simulink model "run_bota_ethercat"  (R2021b)
settings: Solver=ode5  StartTime=0.0  StopTime=inf  FixedStep=0.001  RelTol=1e-3
settings Model: Creator=Martin Wermelinger  LastModifiedBy=Martin Wermelinger
settings CodeAppCC: MaxIdLength=95

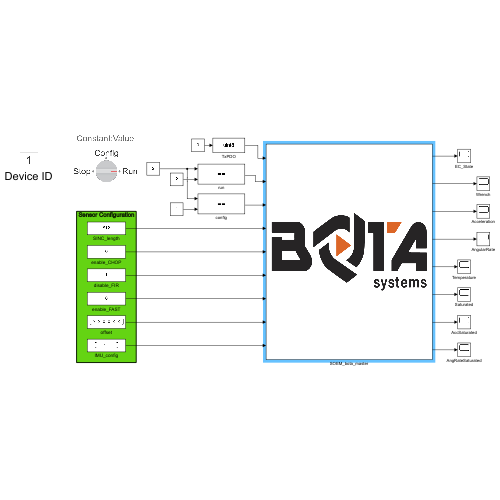
[thumbnail: Simulink's stored preview of the top-level diagram]
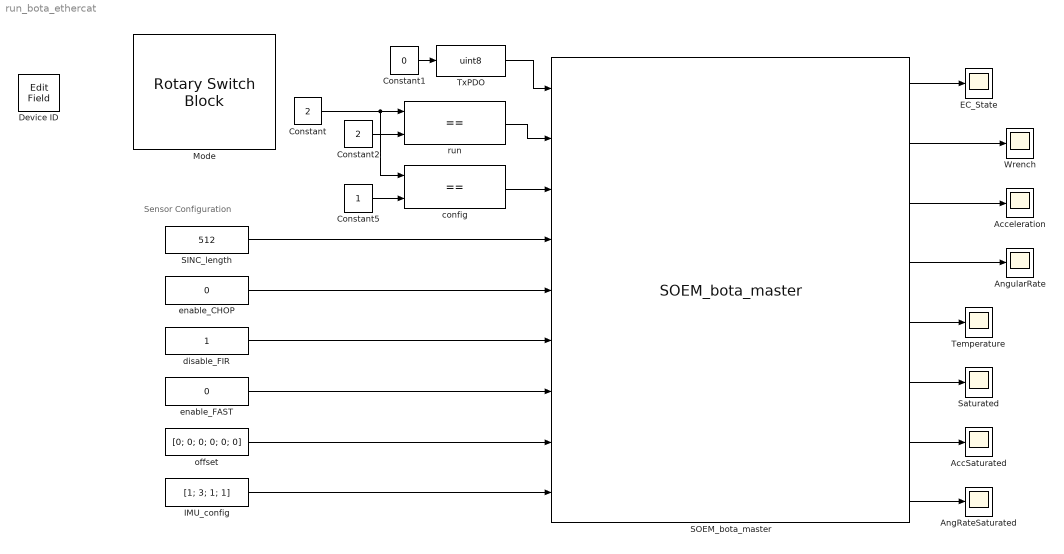
== system run_bota_ethercat ==
  note: Sensor Configuration
  AccSaturated : Scope
  Acceleration : Scope
  AngRateSaturated : Scope
  AngularRate : Scope
  Constant : Constant  Value=2  SampleTime=-1
  Constant1 : Constant  Value=0  SampleTime=0.001
  Constant2 : Constant  Value=2  SampleTime=-1
  Constant5 : Constant  SampleTime=-1
  Device ID : EditField  LabelPosition=Hide  ShowInitialText=on  Alignment=Center
  EC_State : Scope
  IMU_config : Constant  Value=[1; 3; 1; 1]  OutDataTypeStr=int8  SampleTime=-1
  Mode : RotarySwitchBlock
      settings: Values={{'Stop', 'Config', 'Run'}, [-1 1 2]}
  SINC_length : Constant  Value=512  OutDataTypeStr=uint16  SampleTime=-1
  SOEM_bota_master : S-Function  FunctionName=SOEM_bota_master  Parameters=1  SFunctionDeploymentMode=off  EnableBusSupport=off
      mask Display: image('$imagefile'); % Use "Edit Image" on toolstrip to change.
  Saturated : Scope
  Temperature : Scope
  TxPDO : DataTypeConversion  OutDataTypeStr=uint8
  Wrench : Scope
  config : RelationalOperator  Operator===  OutDataTypeStr=boolean  RndMeth=Simplest
  disable_FIR : Constant  OutDataTypeStr=uint8  SampleTime=-1
  enable_CHOP : Constant  Value=0  OutDataTypeStr=uint8  SampleTime=-1
  enable_FAST : Constant  Value=0  OutDataTypeStr=uint8  SampleTime=-1
  offset : Constant  Value=[0; 0; 0; 0; 0; 0]  OutDataTypeStr=single  SampleTime=-1
  run : RelationalOperator  Operator===  OutDataTypeStr=boolean  RndMeth=Simplest
  wires:
  IMU_config/1 -> SOEM_bota_master/9
  TxPDO/1 -> SOEM_bota_master/1
  SOEM_bota_master/1 -> EC_State/1
  offset/1 -> SOEM_bota_master/8
  Constant/1 -> config/1, run/1
  SOEM_bota_master/4 -> AngularRate/1
  SOEM_bota_master/8 -> AngRateSaturated/1
  SOEM_bota_master/7 -> AccSaturated/1
  SOEM_bota_master/6 -> Saturated/1
  SOEM_bota_master/5 -> Temperature/1
  Constant1/1 -> TxPDO/1
  SOEM_bota_master/3 -> Acceleration/1
  run/1 -> SOEM_bota_master/2
  Constant5/1 -> config/2
  disable_FIR/1 -> SOEM_bota_master/6
  enable_CHOP/1 -> SOEM_bota_master/5
  config/1 -> SOEM_bota_master/3
  SINC_length/1 -> SOEM_bota_master/4
  enable_FAST/1 -> SOEM_bota_master/7
  Constant2/1 -> run/2
  SOEM_bota_master/2 -> Wrench/1
